simulink model "shifter_start"  (R2018a)
settings: Solver=FixedStepAuto  StartTime=0.0  StopTime=30  FixedStep=0.05  RelTol=1e-3  EnableMultiTasking=on
settings Model: Creator=jrivitus  LastModifiedBy=Brady
settings DataIOCC: ExternalInput=[t, up_threshold, vehicle_speed, down_threshold]  LimitDataPoints=on  LoadExternalInput=on  SaveFormat=Array
settings OptimizationCC: ExpressionDepthLimit=2147483647  LifeSpan=inf
settings DebuggingCC: UnderspecifiedInitializationDetection=Classic  MergeDetectMultiDrivingBlocksExec=none  ParameterPrecisionLossMsg=none  FcnCallInpInsideContextMsg=warning  AllowSymbolicDim=off  StateNameClashWarn=warning  SFUnexpectedBacktrackingDiag=warning  SFNoUnconditionalDefaultTransitionDiag=warning  SFExecutionAtInitializationDiag=none
settings HardwareCC: ProdBitPerPointer=32  ProdBitPerSizeT=32  ProdBitPerPtrDiffT=32  ProdLargestAtomicFloat=None  ProdIntDivRoundTo=Undefined  ProdEndianess=Unspecified  ProdWordSize=32  ProdHWDeviceType=32-bit Generic
settings ModelReferenceCC: PropagateSignalLabelsOutOfModel=off
settings CodeAppCC: StateflowObjectComments=on
settings GRTTargetCC: TargetLangStandard=C89/C90 (ANSI)  GeneratePreprocessorConditionals=Disable all  CombineOutputUpdateFcns=off  GRTInterface=on
settings ConfigComp: CovMetricSettings=dw  CovHtmlReporting=on  CovSaveCumulativeToWorkspaceVar=on  CovSaveSingleToWorkspaceVar=on  CovExternalEMLEnable=off  CovSFcnEnable=off

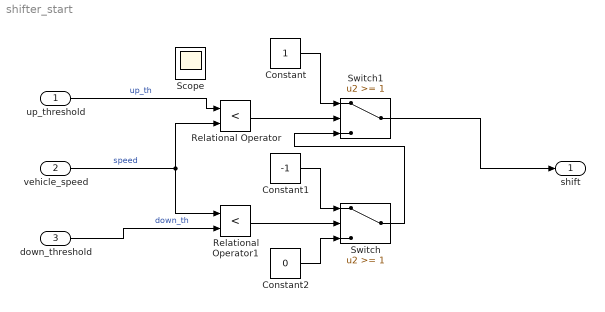
== system shifter_start ==
  up_threshold : Inport  OutDataTypeStr=double
  vehicle_speed : Inport  Port=2  OutDataTypeStr=double
  down_threshold : Inport  Port=3  OutDataTypeStr=double
  Constant : Constant
  Constant1 : Constant  Value=-1
  Constant2 : Constant  Value=0
  Relational Operator : RelationalOperator  Operator=<  OutDataTypeStr=boolean  RndMeth=Simplest
  Relational Operator1 : RelationalOperator  Operator=<  OutDataTypeStr=boolean  RndMeth=Simplest
  Switch : Switch  Threshold=1
  Switch1 : Switch  Threshold=1
  shift : Outport
  Scope : Scope
  wires:
  up_threshold/1 -> Relational Operator/1  "up_th"
  vehicle_speed/1 -> Relational Operator/2, Relational Operator1/1  "speed"
  down_threshold/1 -> Relational Operator1/2  "down_th"
  Relational Operator1/1 -> Switch/2
  Switch/1 -> Switch1/3
  Relational Operator/1 -> Switch1/2
  Constant1/1 -> Switch/1
  Constant2/1 -> Switch/3
  Constant/1 -> Switch1/1
  Switch1/1 -> shift/1
